simulink model "Simulink_Linearization_Model_FMIKit"  (R2022b)
settings: Solver=ode4  StartTime=0.0  StopTime=200  FixedStep=0.001  RelTol=1e-3
undefined symbols (not defined in the file or in its folder): FMIKit
libraries: simulink_extras x1, simulink x1
settings Model: Creator=ka402286  LastModifiedBy=mo780715
settings DataIOCC: SaveState=on
settings OptimizationCC: BlockReduction=off  DefaultParameterBehavior=Inlined  BufferReuse=off
settings ModelReferenceCC: EnableRefExpFcnMdlSchedulingChecks=on
settings RTWCC: RetainRTWFile=on  CustomInclude="\"C:\\Users\\ka402286\\Documents\\PhD Reseacrh\\Fatigue Load reduction Using IPC(By Dq and Atlas Theory)\\Linearization\\FMIKit-Simulink-2.9\\include\" \"C:\\Users\\ka402286\\Documents\\PhD Reseacrh\\Fatigue Load reduction Using IPC(By Dq and Atlas Theory)\\Load Reduction\\FMIKit-Simulink-2.9\\include\" \"C:\\Users\\ka402286\\Documents\\test\\FMIKit-Simulink-2.9\\include\" \"C:\\Users\\ka402286\\Documents\\PhD Reseacrh\\Fatigue load reduction based on RGA\\CRAFTS_Model_at_different_azimuth\\FMIKit-Simulink-2.9\\include\""  CustomSource="\"C:\\Users\\ka402286\\Documents\\PhD Reseacrh\\Fatigue Load reduction Using IPC(By Dq and Atlas Theory)\\Linearization\\FMIKit-Simulink-2.9\\src\\FMU.cpp\" \"C:\\Users\\ka402286\\Documents\\PhD Reseacrh\\Fatigue Load reduction Using IPC(By Dq and Atlas Theory)\\Linearization\\FMIKit-Simulink-2.9\\src\\FMU1.cpp\" \"C:\\Users\\ka402286\\Documents\\PhD Reseacrh\\Fatigue Load reduction Using IPC(By Dq and Atlas Theory)\\Linearization\\FMIKit-Simulink-2.9\\src\\FMU2.cpp\" \"C:\\Users\\ka402286\\Documents\\PhD Reseacrh\\Fatigue Load reduction Using IPC(By Dq and Atlas Theory)\\Load Reduction\\FMIKit-Simulink-2.9\\src\\FMU.cpp\" \"C:\\Users\\ka402286\\Documents\\PhD Reseacrh\\Fatigue Load reduction Using IPC(By Dq and Atlas Theory)\\Load Reduction\\FMIKit-Simulink-2.9\\src\\FMU1.cpp\" \"C:\\Users\\ka402286\\Documents\\PhD Reseacrh\\Fatigue Load reduction Using IPC(By Dq and Atlas Theory)\\Load Reduction\\FMIKit-Simulink-2.9\\src\\FMU2.cpp\" \"C:\\Users\\ka402286\\Documents\\test\\FMIKit-Simulink-2.9\\src\\FMU.cpp\" \"C:\\Users\\ka402286\\Documents\\test\\FMIKit-Simulink-2.9\\src\\FMU1.cpp\" \"C:\\Users\\ka402286\\Documents\\test\\FMIKit-Simulink-2.9\\src\\FMU2.cpp\" \"C:\\Users\\ka402286\\Documents\\PhD Reseacrh\\Fatigue load reduction based on RGA\\CRAFTS_Model_at_different_azimuth\\FMIKit-Simulink-2.9\\src\\FMU.cpp\" \"C:\\Users\\ka402286\\Documents\\PhD Reseacrh\\Fatigue load reduction based on RGA\\CRAFTS_Model_at_different_azimuth\\FMIKit-Simulink-2.9\\src\\FMU1.cpp\" \"C:\\Users\\ka402286\\Documents\\PhD Reseacrh\\Fatigue load reduction based on RGA\\CRAFTS_Model_at_different_azimuth\\FMIKit-Simulink-2.9\\src\\FMU2.cpp\""

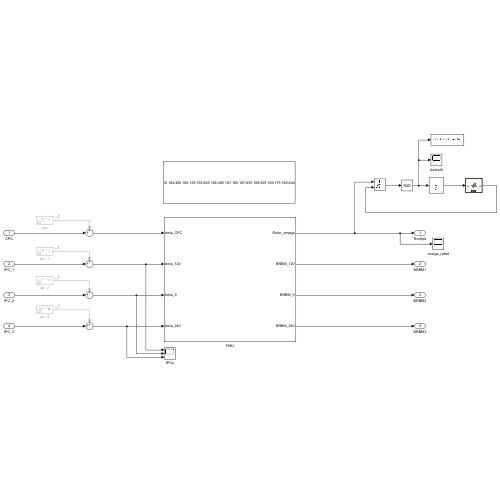
[thumbnail: Simulink's stored preview of the top-level diagram]
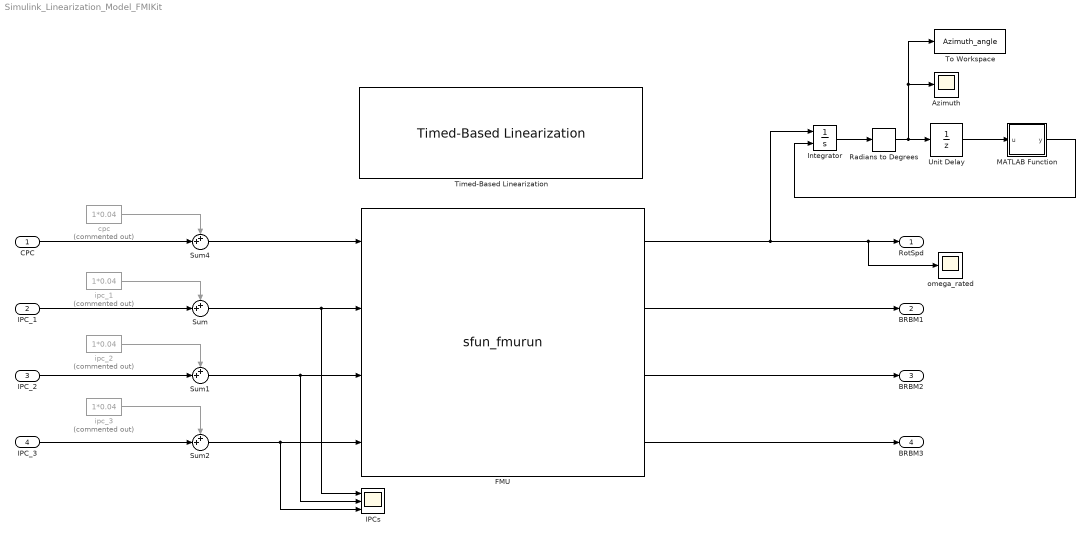
== system Simulink_Linearization_Model_FMIKit ==
  CPC : Inport
  IPC_1 : Inport  Port=2
  IPC_2 : Inport  Port=3
  IPC_3 : Inport  Port=4
  Azimuth : Scope
  FMU : S-Function  LoadFcn=FMIKit.setSFunctionParameters(gcb)  FunctionName=sfun_fmurun  Parameters=2.0 0 '{cb6bfe07-6f6d-49e1-a692-0417e4dd7bac}' 'FMU_QFT_MIMO_Regime3_Simulink_Specific' FMIKit.getUnzipDirectory(gcb) 0 0 0 '' FMIKit.getSolverRelativeTolerance(bdroot(gcb)) -1 0 8 336 0 [1 1 1 1] [1.0 1.0 1.0 1.0] [2 2 2 2] [352321536 352321537 352321538 352321539] [1 1 1 1] [2 2 2 2] [335544320 335544321 335544322 335544323]  SFunctionDeploymentMode=off  EnableBusSupport=off
      settings: DeleteFcn=FMIKit.closeBlockDialog(gcbh)  ModelCloseFcn=FMIKit.closeBlockDialog(gcbh)  DestroyFcn=FMIKit.closeBlockDialog(gcbh)  OpenFcn=FMIKit.showBlockDialog(gcbh);  CloseFcn=FMIKit.closeBlockDialog(gcbh)  ParentCloseFcn=FMIKit.closeBlockDialog(gcbh)
      mask Help: eval('FMIKit.showBlockDialogHelp();')
      mask Display:
      | port_label('input', 1, 'beta_CPC');
      | port_label('input', 2, 'beta_120');
      | port_label('input', 3, 'beta_0');
      | port_label('input', 4, 'beta_240');
      | port_label('output', 1, 'Rotor_omega');
      | port_label('output', 2, 'BRBM_120');
      | port_label('output', 3, 'BRBM_0');
      | port_label('output', 4, 'BRBM_240');
  IPCs : Scope  NumInputPorts=3
  Integrator : Integrator  ExternalReset=rising
  MATLAB Function : MATLAB Function  TreatAsAtomicUnit=on
  Radians to Degrees : simulink_extras/Transformations/Radians to Degrees
  Sum{,1..2,4} (4 alike) : Sum  Inputs=++|
  Timed-Based Linearization : simulink/Model-Wide Utilities/Timed-Based Linearization  LinearizationTime=t_linearization  SampleTime=0
  To Workspace : ToWorkspace  VariableName=Azimuth_angle  SaveFormat=Timeseries  SampleTime=-1
      settings: Decimation=2
  Unit Delay : UnitDelay  SampleTime=-1  HasFrameUpgradeWarning=on
  cpc : Constant  Commented=on  Value=1*0.04
  ipc_1 : Constant  Commented=on  Value=1*0.04
  ipc_2 : Constant  Commented=on  Value=1*0.04
  ipc_3 : Constant  Commented=on  Value=1*0.04
  omega_rated : Scope
  RotSpd : Outport
  BRBM1 : Outport  Port=2
  BRBM2 : Outport  Port=3
  BRBM3 : Outport  Port=4
  wires:
  FMU/2 -> BRBM1/1
  FMU/3 -> BRBM2/1
  FMU/4 -> BRBM3/1
  FMU/1 -> Integrator/1, RotSpd/1, omega_rated/1
  Integrator/1 -> Radians to Degrees/1
  Radians to Degrees/1 -> Azimuth/1, To Workspace/1, Unit Delay/1
  Unit Delay/1 -> MATLAB Function/1(u)
  MATLAB Function/1(y) -> Integrator/2
  ipc_1/1 -> Sum/1
  IPC_1/1 -> Sum/2
  Sum/1 -> FMU/2, IPCs/1
  ipc_2/1 -> Sum1/1
  Sum1/1 -> IPCs/2, FMU/3
  IPC_2/1 -> Sum1/2
  ipc_3/1 -> Sum2/1
  Sum2/1 -> IPCs/3, FMU/4
  IPC_3/1 -> Sum2/2
  Sum4/1 -> FMU/1
  cpc/1 -> Sum4/1
  CPC/1 -> Sum4/2

== matlab function Simulink_Linearization_Model_FMIKit/MATLAB Function ==
  data: u input; y output
function y = fcn(u)
    if u >= 360
        y = 1;
    else
        y = 0;
    end
end
